simulink model "ecc_memory_subsystem"  (R2025b)
settings: Solver=FixedStepDiscrete  StartTime=0.0  StopTime=600  FixedStep=1  RelTol=1e-3
settings Model: Creator=strog  LastModifiedBy=strog

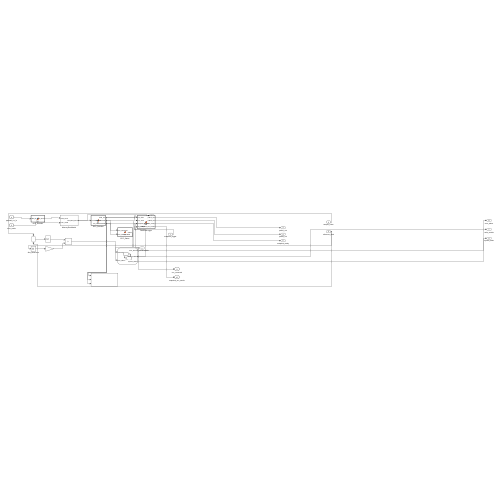
[thumbnail: Simulink's stored preview of the top-level diagram]
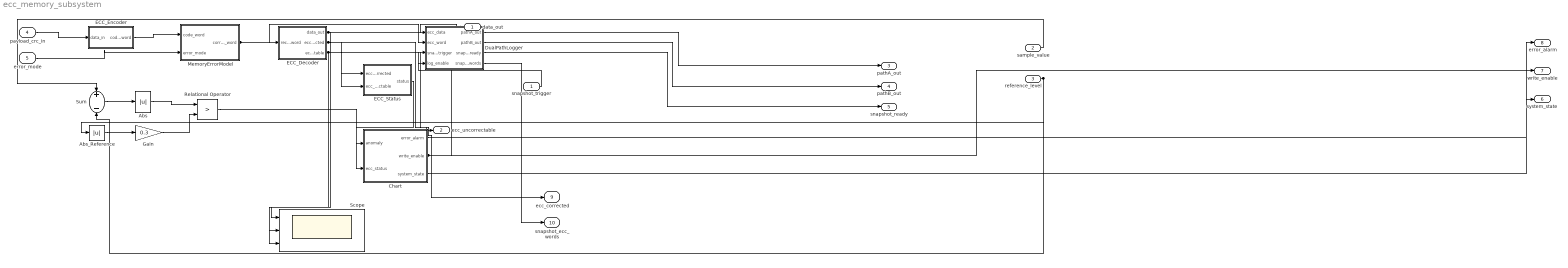
== system ecc_memory_subsystem ==
  snapshot_trigger : Inport  OutDataTypeStr=boolean  PortDimensions=1
  sample_value : Inport  Port=2  OutDataTypeStr=double  PortDimensions=1
  reference_level : Inport  Port=3  OutDataTypeStr=double  PortDimensions=1
  payload_crc_in : Inport  Port=4  OutDataTypeStr=double  PortDimensions=48
  error_mode : Inport  Port=5  OutDataTypeStr=uint8  PortDimensions=1
  Abs : Abs  SaturateOnIntegerOverflow=off
  Abs_Reference : Abs  SaturateOnIntegerOverflow=off
  Chart : Stateflow chart  TreatAsAtomicUnit=on
  DualPathLogger : MATLAB Function  TreatAsAtomicUnit=on
  ECC_Decoder : MATLAB Function  TreatAsAtomicUnit=on
  ECC_Encoder : MATLAB Function  TreatAsAtomicUnit=on
  ECC_Status : MATLAB Function  TreatAsAtomicUnit=on
  Gain : Gain  Gain=0.3
  MemoryErrorModel : Subsystem
  Relational Operator : RelationalOperator  Operator=>  OutDataTypeStr=boolean  RndMeth=Simplest  InputSameDT=off
  Scope : Scope  NumInputPorts=3
      settings: DataLoggingSaveFormat=Array
  Sum : Sum  Inputs=+-
  data_out : Outport
  ecc_uncorrectable : Outport  Port=2
  pathA_out : Outport  Port=3  PortDimensions=48
  pathB_out : Outport  Port=4  PortDimensions=[512 48]
  snapshot_ready : Outport  Port=5
  system_state : Outport  Port=6
  write_enable : Outport  Port=7
  error_alarm : Outport  Port=8
  ecc_corrected : Outport  Port=9
  snapshot_ecc_words : Outport  Port=10  PortDimensions=[512 55]
  wires:
  payload_crc_in/1 -> ECC_Encoder/1(data_in)
  ECC_Encoder/1(code_word) -> MemoryErrorModel/1(code_word)
  error_mode/1 -> MemoryErrorModel/2(error_mode)
  MemoryErrorModel/1(corrupted_word) -> ECC_Decoder/1(received_word), DualPathLogger/2(ecc_word)
  ECC_Decoder/1(data_out) -> data_out/1, DualPathLogger/1(ecc_data), Scope/1
  ECC_Decoder/2(ecc_corrected) -> ecc_corrected/1, ECC_Status/1(ecc_corrected), Scope/2
  ECC_Decoder/3(ecc_uncorrectable) -> ecc_uncorrectable/1, ECC_Status/2(ecc_uncorrectable), Scope/3
  ECC_Status/1(status) -> Chart/2(ecc_status)
  Relational Operator/1 -> Chart/1(anomaly)
  sample_value/1 -> Sum/1
  reference_level/1 -> Sum/2, Abs_Reference/1
  Sum/1 -> Abs/1
  Abs/1 -> Relational Operator/1
  Abs_Reference/1 -> Gain/1
  Gain/1 -> Relational Operator/2
  snapshot_trigger/1 -> DualPathLogger/3(snapshot_trigger)
  Chart/2(write_enable) -> DualPathLogger/4(log_enable), write_enable/1
  DualPathLogger/1(pathA_out) -> pathA_out/1
  DualPathLogger/2(pathB_out) -> pathB_out/1
  DualPathLogger/3(snapshot_ready) -> snapshot_ready/1
  DualPathLogger/4(snapshot_ecc_words) -> snapshot_ecc_words/1
  Chart/1(error_alarm) -> error_alarm/1
  Chart/3(system_state) -> system_state/1

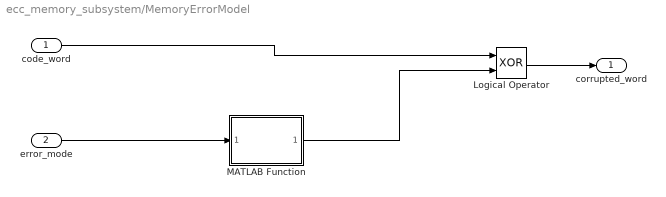
== system ecc_memory_subsystem/MemoryErrorModel ==
  code_word : Inport
  error_mode : Inport  Port=2
  Logical Operator : Logic  Operator=XOR  AllPortsSameDT=off  OutDataTypeStr=boolean
  MATLAB Function : MATLAB Function  TreatAsAtomicUnit=on
  corrupted_word : Outport
  wires:
  code_word/1 -> Logical Operator/1
  error_mode/1 -> MATLAB Function/1(error_mode)
  MATLAB Function/1(error_mask) -> Logical Operator/2
  Logical Operator/1 -> corrupted_word/1

== matlab function ecc_memory_subsystem/ECC_Decoder ==
  data: received_word input size=[1 55]; data_out output size=[1 48]; ecc_corrected output; ecc_uncorrectable output
function [data_out, ecc_corrected, ecc_uncorrectable] = fcn(received_word)
%#codegen
parity_positions = [1 2 4 8 16 32];
data_positions = setdiff(1:54, parity_positions);
r = reshape(double(received_word), 1, 55);
syndrome = 0;
for parity_index = 1:6
    parity_position = parity_positions(parity_index);
    parity_value = 0;
    for bit_position = 1:54
        if bitand(uint32(bit_position), uint32(parity_position)) ~= 0
            parity_value = mod(parity_value + r(bit_position), 2);
        end
    end
    if parity_value ~= 0
        syndrome = syndrome + parity_position;
    end
end
overall_error = mod(sum(r), 2) ~= 0;
ecc_corrected = 0;
ecc_uncorrectable = 0;
if syndrome == 0 && overall_error
    r(55) = 1 - r(55);
    ecc_corrected = 1;
elseif syndrome ~= 0 && overall_error && syndrome <= 54
    r(syndrome) = 1 - r(syndrome);
    ecc_corrected = 1;
elseif syndrome ~= 0 && ~overall_error
    ecc_uncorrectable = 1;
end
data_out = zeros(1, 48);
if ecc_uncorrectable == 0
    data_out = r(data_positions);
end
end

== matlab function ecc_memory_subsystem/ECC_Encoder ==
  data: data_in input size=[1 48]; code_word output size=[1 55]
function code_word = fcn(data_in)
%#codegen
parity_positions = [1 2 4 8 16 32];
data_positions = setdiff(1:54, parity_positions);
code_word = zeros(1, 55);
for data_index = 1:48
    code_word(data_positions(data_index)) = mod(double(data_in(data_index)), 2);
end
for parity_index = 1:6
    parity_position = parity_positions(parity_index);
    parity_value = 0;
    for bit_position = 1:54
        if bitand(uint32(bit_position), uint32(parity_position)) ~= 0
            parity_value = mod(parity_value + code_word(bit_position), 2);
        end
    end
    code_word(parity_position) = parity_value;
end
code_word(55) = mod(sum(code_word(1:54)), 2);
end

== matlab function ecc_memory_subsystem/MemoryErrorModel/MATLAB Function ==
  data: error_mode input; error_mask output size=[1 55]
function error_mask = fcn(error_mode)
%#codegen
error_mask = zeros(1, 55);
if error_mode == 1
    error_mask(5) = 1;
elseif error_mode == 2
    error_mask(5) = 1;
    error_mask(12) = 1;
end
end

== stateflow chart ecc_memory_subsystem/Chart ==
  state Error
    entry:
    write_enable = false;
    error_alarm = true;
    system_state = 5;
  state Normal
    entry:
    write_enable = true;
    error_alarm = false;
    system_state = 1;
  state Snapshot
    entry:
    write_enable = true;
    system_state = 3;
  state RetryECC
    entry:
    write_enable = false;
    system_state = 4;
  state Alarm
    entry:
    anomaly_counter = 0;
    during:
    if anomaly
    anomaly_counter = anomaly_counter + 1;
    else
    anomaly_counter = 0;
    end
    system_state=2;
  (default) -> Normal
  RetryECC -> Error [order 2] : [ecc_status==2]
  RetryECC -> Normal [order 3] : [ecc_status == 0 || (ecc_status == 1 && ~any(anomaly))]
  Alarm -> Normal [order 2] : [~anomaly]
  Normal -> Alarm : [anomaly]
  Snapshot -> RetryECC
  Alarm -> Snapshot [order 1] : [anomaly_counter>=3]
  RetryECC -> Alarm [order 1] : [ecc_status ==1 && any(anomaly)]
  data: anomaly input boolean size=1; ecc_status input uint8 size=1; error_alarm output boolean; write_enable output boolean; anomaly_counter local; system_state output uint8

== matlab function ecc_memory_subsystem/DualPathLogger ==
  data: ecc_data input size=[1 48]; ecc_word input size=[1 55]; pathA_out output size=[1 48]; snapshot_trigger input; log_enable input; pathB_out output size=[512 48]; snapshot_ready output; snapshot_ecc_words output size=[512 55]
function [pathA_out, pathB_out, snapshot_ready, snapshot_ecc_words] = fcn(ecc_data, ecc_word, snapshot_trigger, log_enable)
%#codegen
persistent ring_buffer ring_codewords write_index valid_count snapshot_buffer snapshot_codewords recording post_count previous_trigger
if isempty(ring_buffer)
    ring_buffer = zeros(512, 48);
    ring_codewords = zeros(512, 55);
    write_index = 1;
    valid_count = 0;
    snapshot_buffer = zeros(512, 48);
    snapshot_codewords = zeros(512, 55);
    recording = false;
    post_count = 0;
    previous_trigger = false;
end
snapshot_ready = false;
trigger_active = snapshot_trigger ~= 0;
if log_enable
    if trigger_active && ~previous_trigger && ~recording
        snapshot_buffer = zeros(512, 48);
        snapshot_codewords = zeros(512, 55);
        pre_count = min(valid_count, 256);
        for index = 1:pre_count
            source_index = mod(write_index - pre_count + index - 2, 512) + 1;
            destination_index = 257 - pre_count + index - 1;
            snapshot_buffer(destination_index, :) = ring_buffer(source_index, :);
            snapshot_codewords(destination_index, :) = ring_codewords(source_index, :);
        end
        snapshot_buffer(257, :) = ecc_data;
        snapshot_codewords(257, :) = ecc_word;
        recording = true;
        post_count = 1;
    elseif recording
        if post_count < 256
            post_count = post_count + 1;
            snapshot_buffer(256 + post_count, :) = ecc_data;
            snapshot_codewords(256 + post_count, :) = ecc_word;
        end
        if post_count == 256
            recording = false;
            snapshot_ready = true;
        end
    end
    ring_buffer(write_index, :) = ecc_data;
    ring_codewords(write_index, :) = ecc_word;
    write_index = mod(write_index, 512) + 1;
    valid_count = min(valid_count + 1, 512);
end
previous_trigger = trigger_active;
pathA_out = zeros(1, 48);
if log_enable
    pathA_out = ecc_data;
end
pathB_out = snapshot_buffer;
snapshot_ecc_words = snapshot_codewords;
end

== matlab function ecc_memory_subsystem/ECC_Status ==
  data: ecc_corrected input; status output; ecc_uncorrectable input
function status = fcn(ecc_corrected, ecc_uncorrectable)
%#codegen
status = uint8(0);
if ecc_uncorrectable ~= 0
    status = uint8(2);
elseif ecc_corrected ~= 0
    status = uint8(1);
end
end
